simulink model "uravnenie_zadacha"  (Simulink 6.3)
settings: Solver=ode45  StartTime=0.0  StopTime=10.0  RelTol=1e-3
undefined symbols (not defined in the file): magnitude
libraries: simulink x1
settings Model: LastModifiedBy=Ms1

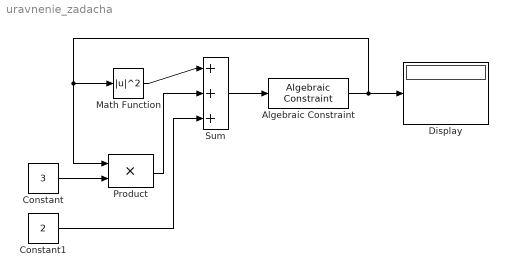
== system uravnenie_zadacha ==
  Algebraic Constraint : simulink/Math Operations/Algebraic Constraint  z0=[0 -3]
  Constant : Constant  Value=3
  Constant1 : Constant  Value=2
  Display : Display
  Math Function : Math  Operator=magnitude^2  SaturateOnIntegerOverflow=on
  Product : Product  SaturateOnIntegerOverflow=on  InputSameDT=on
  Sum : Sum  Inputs=|+++  SaturateOnIntegerOverflow=on  InputSameDT=on
  wires:
  Algebraic Constraint/1 -> Math Function/1, Product/1, Display/1
  Math Function/1 -> Sum/1
  Sum/1 -> Algebraic Constraint/1
  Constant/1 -> Product/2
  Product/1 -> Sum/2
  Constant1/1 -> Sum/3
